simulink subsystem "RateModulation"  (R2022a)
settings: Solver=VariableStepAuto  StartTime=0.0  StopTime=10.0  RelTol=1e-3
settings Model: Creator=bkfre  LastModifiedBy=bkfre

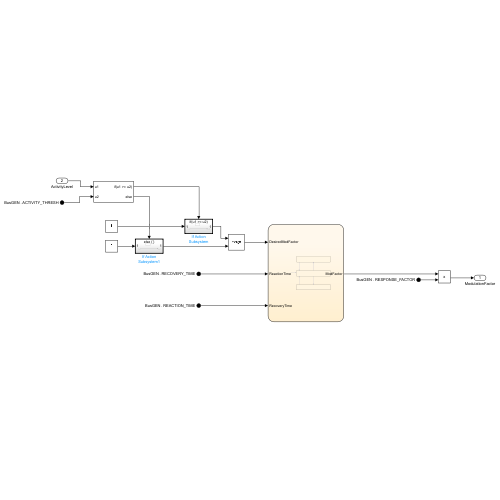
[thumbnail: Simulink's stored preview of the top-level diagram]
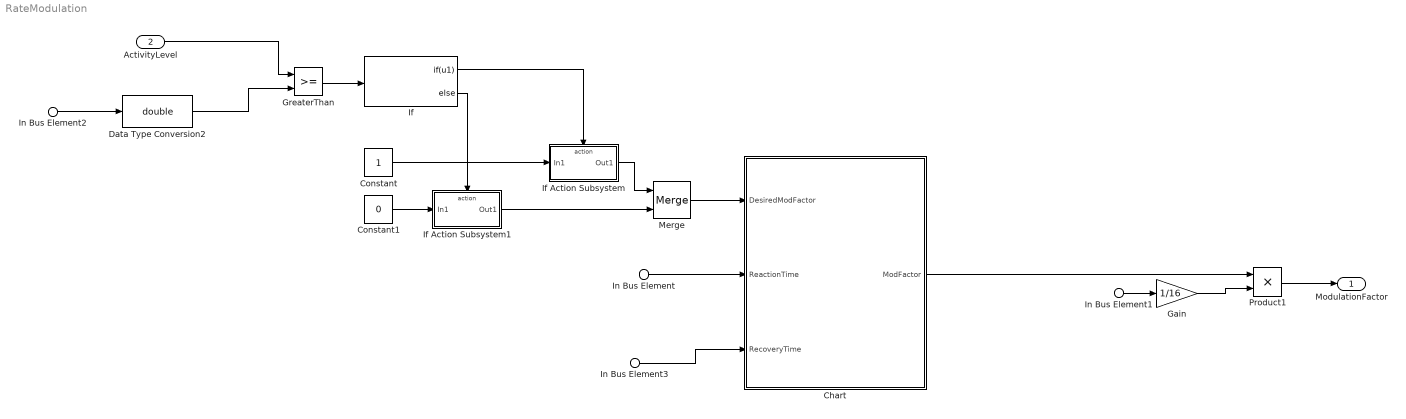
== system RateModulation ==
  In Bus Element2 : Inport  PortName=BusGEN  Element=ACTIVITY_THRESH
  In Bus Element : Inport  PortName=BusGEN  Element=REACTION_TIME
  In Bus Element1 : Inport  PortName=BusGEN  Element=RESPONSE_FACTOR
  In Bus Element3 : Inport  PortName=BusGEN  Element=RECOVERY_TIME
  ActivityLevel : Inport  Port=2
  Chart : Stateflow chart  TreatAsAtomicUnit=on
      settings: PortSchema="{\"entries\":[{\"content\":{\"sides\":[{\"content\":{\"connectorIds\":[\"In3\",\"In1\",\"In2\"]},\"type\":\"ConnectorPlacement.EquallySpacedRectSide\",\"uuid\":\"513776f1-3486-4818-b039-03cfe09a19f1\"},{\"content\":{\"connectorIds\":[\"Out1\"],\"side\":\"RIGHT\"},\"type\":\"ConnectorPlacement.EquallySpacedRectSide\",\"uuid\":\"f9256409-ae31-46ca-b6f9-711c202b9689\"},{\"content\":{\"connectorIds\":[],\"side\":\"TOP\"},\"type\":\"ConnectorPlacement.EquallySpacedRectSide\",\"uuid\":\"f4558c9f-6405-4a5b-af0e-1816af9fa287\"}]},\"type\":\"ConnectorPlacement.EquallySpacedConnector\",\"uuid\":\"7f505aeb-9e7d-4efc-b380-7acb9d8ef140\"}],\"packageUris\":[\"http://schema.mathworks.com/mf0/Connector/R2020b\"],\"version\":\"1.0\"}"
  Constant : Constant  OutDataTypeStr=double
  Constant1 : Constant  Value=0  OutDataTypeStr=double
  Data Type Conversion2 : DataTypeConversion  OutDataTypeStr=double  SaturateOnIntegerOverflow=off  RndMeth=Floor
  Gain : Gain  Gain=1/16
  GreaterThan : RelationalOperator  OutDataTypeStr=boolean  RndMeth=Simplest  InputSameDT=off
  If : If  IfExpression=u1
  If Action Subsystem : Subsystem  TreatAsAtomicUnit=on
  If Action Subsystem1 : Subsystem  TreatAsAtomicUnit=on
  Merge : Merge
  Product1 : Product
  ModulationFactor : Outport
  wires:
  Chart/1(ModFactor) -> Product1/1
  Product1/1 -> ModulationFactor/1
  Merge/1 -> Chart/3(DesiredModFactor)
  Constant/1 -> If Action Subsystem/1(In1)
  Constant1/1 -> If Action Subsystem1/1(In1)
  If Action Subsystem1/1(Out1) -> Merge/2
  If Action Subsystem/1(Out1) -> Merge/1
  If/1 -> If Action Subsystem/Action
  If/2 -> If Action Subsystem1/Action
  In Bus Element3/1 -> Chart/2(RecoveryTime)
  In Bus Element1/1 -> Gain/1
  In Bus Element2/1 -> Data Type Conversion2/1
  GreaterThan/1 -> If/1
  ActivityLevel/1 -> GreaterThan/1
  Gain/1 -> Product1/2
  In Bus Element/1 -> Chart/1(ReactionTime)
  Data Type Conversion2/1 -> GreaterThan/2

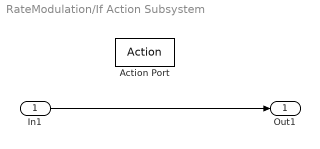
== system RateModulation/If Action Subsystem ==
  In1 : Inport
  Action Port : ActionPort
  Out1 : Outport
  wires:
  In1/1 -> Out1/1

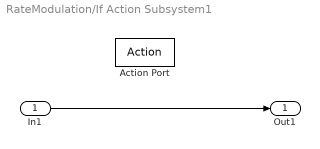
== system RateModulation/If Action Subsystem1 ==
  In1 : Inport
  Action Port : ActionPort
  Out1 : Outport
  wires:
  In1/1 -> Out1/1

== stateflow chart RateModulation/Chart ==
  state SpeedUp
    during:
    ModFactor = ModFactor + 0.001 / ReactionTime;
  state Hold
  state SlowDown
    during:
    ModFactor = ModFactor - 0.001 / (RecoveryTime * 60);
  SpeedUp -> Hold : [DesiredModFactor <= ModFactor]
  Hold -> SpeedUp [order 1] : [DesiredModFactor > ModFactor + 0.01]
  (default) -> Hold
  SlowDown -> Hold : [DesiredModFactor >= ModFactor]
  Hold -> SlowDown [order 2] : [DesiredModFactor < ModFactor - 0.01]
  data: ReactionTime input; RecoveryTime input; DesiredModFactor input; ModFactor output =0
